simulink model "LazosdeCorriente"  (R2023b)
settings: Solver=VariableStepAuto  StartTime=0.0  StopTime=10.0  RelTol=1e-3
values from neighbouring files (symbols this model uses):
  L_d = 6.6 * 10^(-3)    (= 0.0066)    [varLC.m]
  lambda_m = 0.016    [varLC.m]
  P_p = 3    [Controlador.m]    (also in varLC.m)
  R_0 = 4    [varLC.m]
  R_d = 33    [varLC.m]
  R_q = 29    [varLC.m]
settings Model: Creator=tomas  LastModifiedBy=gonza

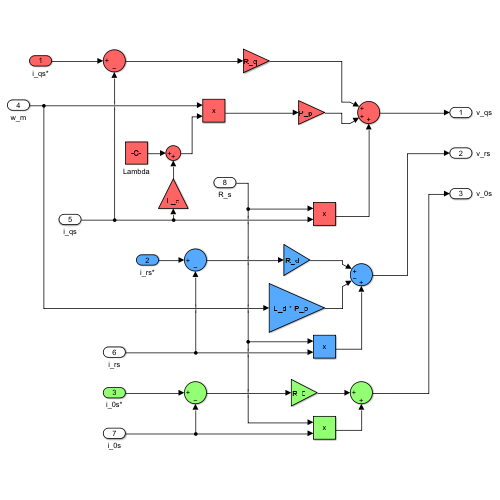
[thumbnail: Simulink's stored preview of the top-level diagram]
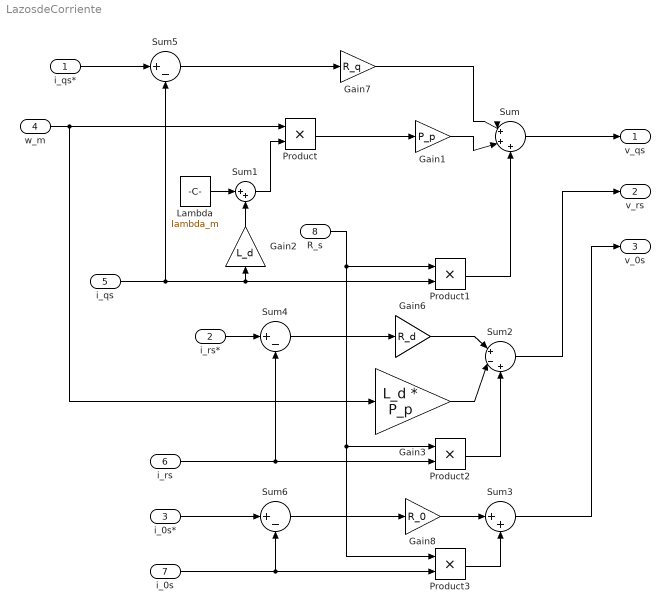
== system LazosdeCorriente ==
  i_qs* : Inport
  i_rs* : Inport  Port=2
  i_0s* : Inport  Port=3
  w_m : Inport  Port=4
  i_qs : Inport  Port=5
  i_rs : Inport  Port=6
  i_0s : Inport  Port=7
  R_s : Inport  Port=8
  Gain1 : Gain  Gain=P_p
  Gain2 : Gain  Gain=L_d
  Gain3 : Gain  Gain=L_d * P_p
  Gain6 : Gain  Gain=R_d
  Gain7 : Gain  Gain=R_q
  Gain8 : Gain  Gain=R_0
  Lambda : Constant  Value=lambda_m
  Product{,1..3} (4 alike) : Product
  Sum : Sum  Inputs=|+++
  Sum1 : Sum  Inputs=|++
  Sum2 : Sum  Inputs=|+-+
  Sum3 : Sum  Inputs=|++
  Sum4 : Sum  Inputs=|+-
  Sum5 : Sum  Inputs=|+-
  Sum6 : Sum  Inputs=|+-
  v_qs : Outport
  v_rs : Outport  Port=2
  v_0s : Outport  Port=3
  wires:
  i_rs/1 -> Product2/2, Sum4/2
  Gain1/1 -> Sum/2
  w_m/1 -> Gain3/1, Product/1
  Lambda/1 -> Sum1/1
  Gain2/1 -> Sum1/2
  Sum1/1 -> Product/2
  Product/1 -> Gain1/1
  Sum/1 -> v_qs/1
  Gain3/1 -> Sum2/2
  Product2/1 -> Sum2/3
  Product3/1 -> Sum3/2
  i_0s/1 -> Product3/2, Sum6/2
  Sum3/1 -> v_0s/1
  Sum2/1 -> v_rs/1
  i_rs*/1 -> Sum4/1
  Sum4/1 -> Gain6/1
  Gain6/1 -> Sum2/1
  i_qs/1 -> Sum5/2, Product1/2, Gain2/1
  i_qs*/1 -> Sum5/1
  Sum5/1 -> Gain7/1
  Gain7/1 -> Sum/1
  i_0s*/1 -> Sum6/1
  Sum6/1 -> Gain8/1
  Gain8/1 -> Sum3/1
  Product1/1 -> Sum/3
  R_s/1 -> Product3/1, Product2/1, Product1/1
